simulink model "bike_model_pidTuning"  (R2018b)
settings: Solver=FixedStepAuto  StartTime=0.0  StopTime=sim_time  FixedStep=Ts_IMU  MaxStep=Ts  RelTol=1e-3
values from neighbouring files (symbols this model uses):
  a_compFilter = b_compFilter - 0.77    (= 0.325)    [configuration.m]
  b_compFilter = 1.095    [configuration.m]
  b_real = 1.095    [configuration.m]
  direct_control = 1    [configuration.m]
  IMU_height_real = 0.45    [configuration.m]
  initial_states = [deg2rad(-2) deg2rad(0) deg2rad(0)]    [configuration.m]
  input_velocity = 3    [configuration.m]
  lambda_compFilter = deg2rad(70)    [configuration.m]
  lambda_real = deg2rad(70)    [configuration.m]
  look_ahead = 0    [configuration.m]
  parameters_compFilter = [g h_compFilter b_compFilter a_compFilter lambda_compFilter c_compFilter]    [configuration.m]
  parameters_f_b_real = [m_frame_real m_box_real h_frame_real h_box_real a_frame_real a_box_real c_frame_real c_box_real b_frame_real b_box_real l_frame_real l_box_real]    [configuration.m]
  parameters_real = [g h_real b_real a_real lambda_real c_real]    [configuration.m]
  plant_model = 1    [configuration.m]
  Ts = 0.04    [configuration.m]
  Ts_IMU = 0.04    [configuration.m]
undefined symbols (not defined in the file or in its folder): cumulative_dist_along_path, curvature, DiscIntNeverNeededParam, initial_x, initial_y, lqr_gains, path_x, path_y, sys_con, sys_dis, velocity_lqr
libraries: simulink x20, dspsigops x2
(part 1 of 2)
settings Model: Creator=Boaz Ash  LastModifiedBy=maximef
settings DebuggingCC: UnconnectedInputMsg=none  UnconnectedOutputMsg=none  UnconnectedLineMsg=none  LibraryContextMissingDiagnostic=none
settings SFSimCC: SimUseLocalCustomCode=off
settings RTWCC: RTWUseLocalCustomCode=off

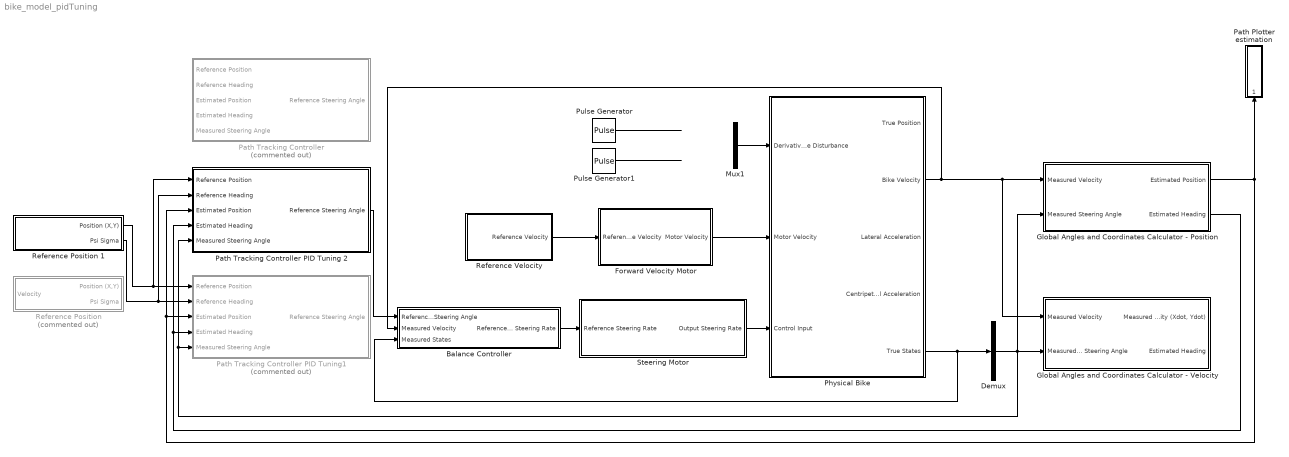
== system bike_model_pidTuning ==
  Balance Controller : Subsystem  TreatAsAtomicUnit=on  SystemSampleTime=Ts
  Demux : Demux  Outputs=3
  Forward Velocity Motor : Subsystem
  Global Angles and Coordinates Calculator - Position : Subsystem  SystemSampleTime=Ts
  Global Angles and Coordinates Calculator - Velocity : Subsystem  SystemSampleTime=Ts
  Mux1 : Mux  Inputs=3
  Path Plotter estimation : Subsystem  SystemSampleTime=Ts
  Path Tracking Controller : Subsystem  Commented=on
  Path Tracking Controller PID Tuning 2 : Subsystem
  Path Tracking Controller PID Tuning1 : Subsystem  Commented=on
  Physical Bike : Subsystem
  Pulse Generator : DiscretePulseGenerator  PulseType=Time based  Amplitude=pi/36  Period=100  PhaseDelay=1
  Pulse Generator1 : DiscretePulseGenerator  PulseType=Time based  Amplitude=-deg2rad(30)  Period=10  PulseWidth=10  PhaseDelay=1
  "Reference Position " : Subsystem  Commented=on
  Reference Position 1 : Subsystem
  "Reference Velocity " : Subsystem
  Steering Motor : Subsystem
  wires:
  Pulse Generator/1 -> ?
  Pulse Generator1/1 -> ?
  Physical Bike/2(Bike Velocity) -> Balance Controller/2(Measured Velocity), Global Angles and Coordinates Calculator - Velocity/1(Measured Velocity), Global Angles and Coordinates Calculator - Position/1(Measured Velocity)
  Reference Position 1/1(Position (X,Y)) -> Path Tracking Controller PID Tuning 2/1(Reference Position), Path Tracking Controller PID Tuning1/1(Reference Position)
  Path Tracking Controller PID Tuning 2/1(Reference Steering Angle) -> Balance Controller/1(Reference Steering Angle)
  Forward Velocity Motor/1(Motor Velocity) -> Physical Bike/2(Motor Velocity)
  Reference Position 1/2(Psi Sigma) -> Path Tracking Controller PID Tuning 2/2(Reference Heading), Path Tracking Controller PID Tuning1/2(Reference Heading)
  "Reference Velocity "/1(Reference Velocity) -> Forward Velocity Motor/1(Reference Velocity)
  Steering Motor/1(Output Steering Rate) -> Physical Bike/3(Control Input)
  Balance Controller/1(Reference Steering Rate) -> Steering Motor/1(Reference Steering Rate)
  Physical Bike/5(True States) -> Balance Controller/3(Measured States), Demux/1
  Global Angles and Coordinates Calculator - Position/2(Estimated Heading) -> Path Tracking Controller PID Tuning 2/4(Estimated Heading), Path Tracking Controller PID Tuning1/4(Estimated Heading)
  Demux/2 -> Global Angles and Coordinates Calculator - Velocity/2("Measured Steering Angle "), Global Angles and Coordinates Calculator - Position/2(Measured Steering Angle), Path Tracking Controller PID Tuning 2/5(Measured Steering Angle), Path Tracking Controller PID Tuning1/5(Measured Steering Angle)
  Mux1/1 -> Physical Bike/1(Derivative Disturbance)
  Global Angles and Coordinates Calculator - Position/1(Estimated Position) -> Path Plotter estimation/1(Position), Path Tracking Controller PID Tuning 2/3(Estimated Position), Path Tracking Controller PID Tuning1/3(Estimated Position)

== system bike_model_pidTuning/Balance Controller ==
  Reference Steering Angle : Inport
  Measured Velocity : Inport  Port=2
  Measured States : Inport  Port=3
  LQR Controller : Subsystem  TreatAsAtomicUnit=on  SystemSampleTime=Ts
  Reference States : Subsystem  SystemSampleTime=Ts
  Sum : Sum  Inputs=|+-
  To Workspace : ToWorkspace  VariableName=states_measured  SaveFormat=Timeseries  SampleTime=-1
  Reference Steering Rate : Outport
  wires:
  Reference States/1(Reference States) -> Sum/1
  Sum/1 -> LQR Controller/2(State Error)
  LQR Controller/1(Calculated Input) -> Reference Steering Rate/1
  Reference Steering Angle/1 -> Reference States/2(Delta Ref)
  Measured Velocity/1 -> Reference States/1(Velocity), LQR Controller/1(Velocity)
  Measured States/1 -> To Workspace/1, Sum/2

== system bike_model_pidTuning/Forward Velocity Motor ==
  note: Add limit for acceleration/deceleration
      | Add min speed of 1.69 m/s (3600 rpm motor speed) limitation
      | Add min speed of 8.20 m/s (18000 rpm motor speed) limitation
      | Add deadband and delay
  Reference Velocity : Inport
  Motor Velocity : Outport
  wires:
  Reference Velocity/1 -> Motor Velocity/1

== system bike_model_pidTuning/Global Angles and Coordinates Calculator - Position ==
  note: True Steering
      | Angle
  Measured Velocity : Inport
  Measured Steering Angle : Inport  Port=2
  Gain1 : Gain  Gain=sin(lambda_compFilter)
  Measured Bike Angles to Global Angles : Subsystem
  Measured Global Angles to Global Coordinates : Subsystem
  Sum : Sum  Inputs=++|
  Estimated Position : Outport
  Estimated Heading : Outport  Port=2
  wires:
  Measured Bike Angles to Global Angles/1(Psi) -> Sum/2, Measured Global Angles to Global Coordinates/2(Psi)
  Gain1/1 -> Measured Bike Angles to Global Angles/2(Measured Steering Angle)
  Sum/1 -> Estimated Heading/1
  Measured Bike Angles to Global Angles/2(Beta) -> Sum/1, Measured Global Angles to Global Coordinates/3(Beta)
  Measured Global Angles to Global Coordinates/1("Position (X, Y)") -> Estimated Position/1
  Measured Velocity/1 -> Measured Global Angles to Global Coordinates/1(Velocity), Measured Bike Angles to Global Angles/1(Velocity)
  Measured Steering Angle/1 -> Gain1/1

== system bike_model_pidTuning/Global Angles and Coordinates Calculator - Velocity ==
  Measured Velocity : Inport
  "Measured Steering Angle " : Inport  Port=2
  Discrete-Time Integrator : DiscreteIntegrator  SampleTime=-1  ICPrevOutput=DiscIntNeverNeededParam  ICPrevScaledInput=DiscIntNeverNeededParam
  Gain1 : Gain  Gain=sin(lambda_compFilter)
  Measured Bike Angles to Global Angles : Subsystem
  Measured Global Angles to Global Coordinates : Subsystem
  Sum : Sum  Inputs=++|
  To Workspace1 : ToWorkspace  VariableName=pos_vel_int  SaveFormat=Timeseries  SampleTime=-1
  "Measured Velocity (Xdot, Ydot)" : Outport
  Estimated Heading : Outport  Port=2
  wires:
  "Measured Steering Angle "/1 -> Gain1/1
  Measured Bike Angles to Global Angles/1(Psi) -> Sum/2, Measured Global Angles to Global Coordinates/2(Psi)
  Gain1/1 -> Measured Bike Angles to Global Angles/2(Measured Steering Angle)
  Sum/1 -> Estimated Heading/1
  Measured Bike Angles to Global Angles/2(Beta) -> Measured Global Angles to Global Coordinates/3(Beta), Sum/1
  Measured Velocity/1 -> Measured Bike Angles to Global Angles/1(Velocity), Measured Global Angles to Global Coordinates/1(Velocity)
  Measured Global Angles to Global Coordinates/1("Velocity (Xdot, Ydot)") -> "Measured Velocity (Xdot, Ydot)"/1, Discrete-Time Integrator/1
  Discrete-Time Integrator/1 -> To Workspace1/1

== system bike_model_pidTuning/Path Plotter estimation ==
  Position : Inport
  Demux : Demux  Outputs=2
  To Workspace : ToWorkspace  VariableName=X_BIKE_estim  SaveFormat=Timeseries  SampleTime=Ts
  To Workspace1 : ToWorkspace  VariableName=Y_BIKE_estim  SaveFormat=Timeseries  SampleTime=Ts
  XY Graph : simulink/Sinks/XY Graph  Commented=on  xmin=min(path_x)-5  xmax=max(path_x)+5  ymin=min(path_y)-5  ymax=max(path_y)+5  st=-1
  wires:
  Demux/1 -> XY Graph/1, To Workspace/1  "X"
  Demux/2 -> XY Graph/2, To Workspace1/1  "Y"
  Position/1 -> Demux/1

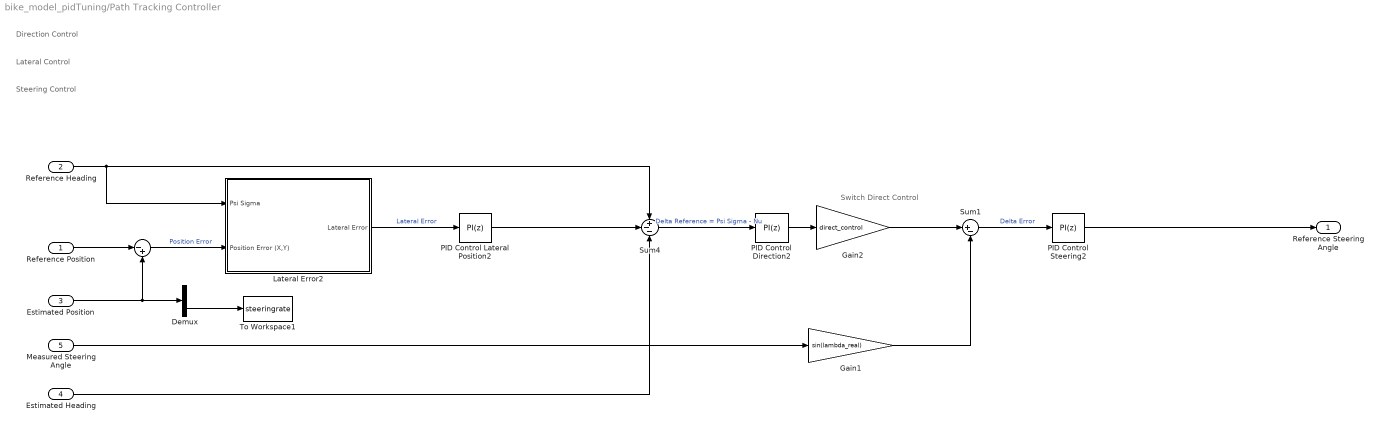
== system bike_model_pidTuning/Path Tracking Controller ==
  note: Direction Control
  note: Lateral Control
  note: Steering Control
  note: Switch Direct Control
  Reference Position : Inport
  Reference Heading : Inport  Port=2
  Estimated Position : Inport  Port=3
  Estimated Heading : Inport  Port=4
  Measured Steering Angle : Inport  Port=5
  " " : Sum  Inputs=|-+
  Demux : Demux  Outputs=2
  Gain1 : Gain  Gain=sin(lambda_real)
  Gain2 : Gain  Gain=direct_control
  Lateral Error2 : Subsystem  SystemSampleTime=Ts
  PID Control Lateral Position2 : simulink/Continuous/PID Controller  Controller=PI  Form=Parallel  TimeDomain=Discrete-time  SampleTime=Ts  IntegratorMethod=Forward Euler  FilterMethod=Forward Euler  ControllerParametersSource=internal  P=0.0465435246389258  I=0.000115580509653549  D=0  UseFilter=on  N=100  TunerSelectOption=Transfer Function Based (PID Tuner App)  InitialConditionSource=internal  InitialConditionForIntegrator=0  InitialConditionForFilter=0  DifferentiatorICPrevScaledInput=0  ExternalReset=none  TrackingMode=off  Kt=1  LimitOutput=off  UpperSaturationLimit=inf  LowerSaturationLimit=-inf  LinearizeAsGain=on  AntiWindupMode=none  Kb=1  POutMin=[]  POutMax=[]  IOutMin=[]  IOutMax=[]  DOutMin=[]  DOutMax=[]  NOutMin=[]  NOutMax=[]  SumOutMin=[]  SumOutMax=[]  SaturationOutMin=[]  SaturationOutMax=[]  PParamMin=[]  PParamMax=[]  IParamMin=[]  IParamMax=[]  DParamMin=[]  DParamMax=[]  NParamMin=[]  NParamMax=[]  KbParamMin=[]  KbParamMax=[]  KtParamMin=[]  KtParamMax=[]  KbOutMin=[]  KbOutMax=[]  KtOutMin=[]  KtOutMax=[]  IntegratorOutMin=[]  IntegratorOutMax=[]  FilterOutMin=[]  FilterOutMax=[]  SumI1OutMin=[]  SumI1OutMax=[]  SumI2OutMin=[]  SumI2OutMax=[]  SumI3OutMin=[]  SumI3OutMax=[]  SumI4OutMin=[]  SumI4OutMax=[]  SumDOutMin=[]  SumDOutMax=[]  DifferentiatorOutMin=[]  DifferentiatorOutMax=[]  FilterDiffOutCoefMin=[]  FilterDiffOutCoefMax=[]  ReciprocalOutMin=[]  ReciprocalOutMax=[]  SumDenOutMin=[]  SumDenOutMax=[]  SumNumOutMin=[]  SumNumOutMax=[]  DivideOutMin=[]  DivideOutMax=[]  IntegratorContinuousStateAttributes=''  IntegratorStateMustResolveToSignalObject=off  IntegratorRTWStateStorageClass=Auto  FilterContinuousStateAttributes=''  FilterStateMustResolveToSignalObject=off  FilterRTWStateStorageClass=Auto  ParallelPVariant=InternalParameters  IdealPVariant=Disabled  IVariant=InternalParameters  DVariant=Disabled  IntegratorVariant=Discrete  SatVariant=Disabled  AWVariant=Passthrough  PCopyVariant=Disabled  TRVariant=Disabled  FdbkBlocksVariant=Forward  IdealPFdbkVariant=Disabled  SatFdbkVariant=Disabled  DerivativeFilterVariant=Disabled  NVariant=Disabled  NCopyVariant=Disabled_SignalSpec  FilterICVariant=Disabled  IntegratorICVariant=InternalICs  ExternalResetVariant=Disabled  TRSumVariant=Passthrough  SumFdbkVariant=Disabled  SumVariant=Sum_PI
  PID Control Direction2 : simulink/Continuous/PID Controller  Controller=PI  Form=Parallel  TimeDomain=Discrete-time  SampleTime=Ts  IntegratorMethod=Forward Euler  FilterMethod=Forward Euler  ControllerParametersSource=internal  P=0.126067479140802  I=0.000739995118675849  D=0  UseFilter=on  N=100  TunerSelectOption=Transfer Function Based (PID Tuner App)  InitialConditionSource=internal  InitialConditionForIntegrator=0  InitialConditionForFilter=0  DifferentiatorICPrevScaledInput=0  ExternalReset=none  TrackingMode=off  Kt=1  LimitOutput=off  UpperSaturationLimit=inf  LowerSaturationLimit=-inf  LinearizeAsGain=on  AntiWindupMode=none  Kb=1  POutMin=[]  POutMax=[]  IOutMin=[]  IOutMax=[]  DOutMin=[]  DOutMax=[]  NOutMin=[]  NOutMax=[]  SumOutMin=[]  SumOutMax=[]  SaturationOutMin=[]  SaturationOutMax=[]  PParamMin=[]  PParamMax=[]  IParamMin=[]  IParamMax=[]  DParamMin=[]  DParamMax=[]  NParamMin=[]  NParamMax=[]  KbParamMin=[]  KbParamMax=[]  KtParamMin=[]  KtParamMax=[]  KbOutMin=[]  KbOutMax=[]  KtOutMin=[]  KtOutMax=[]  IntegratorOutMin=[]  IntegratorOutMax=[]  FilterOutMin=[]  FilterOutMax=[]  SumI1OutMin=[]  SumI1OutMax=[]  SumI2OutMin=[]  SumI2OutMax=[]  SumI3OutMin=[]  SumI3OutMax=[]  SumI4OutMin=[]  SumI4OutMax=[]  SumDOutMin=[]  SumDOutMax=[]  DifferentiatorOutMin=[]  DifferentiatorOutMax=[]  FilterDiffOutCoefMin=[]  FilterDiffOutCoefMax=[]  ReciprocalOutMin=[]  ReciprocalOutMax=[]  SumDenOutMin=[]  SumDenOutMax=[]  SumNumOutMin=[]  SumNumOutMax=[]  DivideOutMin=[]  DivideOutMax=[]  IntegratorContinuousStateAttributes=''  IntegratorStateMustResolveToSignalObject=off  IntegratorRTWStateStorageClass=Auto  FilterContinuousStateAttributes=''  FilterStateMustResolveToSignalObject=off  FilterRTWStateStorageClass=Auto  ParallelPVariant=InternalParameters  IdealPVariant=Disabled  IVariant=InternalParameters  DVariant=Disabled  IntegratorVariant=Discrete  SatVariant=Disabled  AWVariant=Passthrough  PCopyVariant=Disabled  TRVariant=Disabled  FdbkBlocksVariant=Forward  IdealPFdbkVariant=Disabled  SatFdbkVariant=Disabled  DerivativeFilterVariant=Disabled  NVariant=Disabled  NCopyVariant=Disabled_SignalSpec  FilterICVariant=Disabled  IntegratorICVariant=InternalICs  ExternalResetVariant=Disabled  TRSumVariant=Passthrough  SumFdbkVariant=Disabled  SumVariant=Sum_PI
  PID Control Steering2 : simulink/Continuous/PID Controller  Controller=PI  Form=Parallel  TimeDomain=Discrete-time  SampleTime=Ts  IntegratorMethod=Forward Euler  FilterMethod=Forward Euler  ControllerParametersSource=internal  P=0.219020351848633  I=0.4510120195392  D=0  UseFilter=on  N=100  TunerSelectOption=Transfer Function Based (PID Tuner App)  InitialConditionSource=internal  InitialConditionForIntegrator=0  InitialConditionForFilter=0  DifferentiatorICPrevScaledInput=0  ExternalReset=none  TrackingMode=off  Kt=1  LimitOutput=off  UpperSaturationLimit=inf  LowerSaturationLimit=-inf  LinearizeAsGain=on  AntiWindupMode=none  Kb=1  POutMin=[]  POutMax=[]  IOutMin=[]  IOutMax=[]  DOutMin=[]  DOutMax=[]  NOutMin=[]  NOutMax=[]  SumOutMin=[]  SumOutMax=[]  SaturationOutMin=[]  SaturationOutMax=[]  PParamMin=[]  PParamMax=[]  IParamMin=[]  IParamMax=[]  DParamMin=[]  DParamMax=[]  NParamMin=[]  NParamMax=[]  KbParamMin=[]  KbParamMax=[]  KtParamMin=[]  KtParamMax=[]  KbOutMin=[]  KbOutMax=[]  KtOutMin=[]  KtOutMax=[]  IntegratorOutMin=[]  IntegratorOutMax=[]  FilterOutMin=[]  FilterOutMax=[]  SumI1OutMin=[]  SumI1OutMax=[]  SumI2OutMin=[]  SumI2OutMax=[]  SumI3OutMin=[]  SumI3OutMax=[]  SumI4OutMin=[]  SumI4OutMax=[]  SumDOutMin=[]  SumDOutMax=[]  DifferentiatorOutMin=[]  DifferentiatorOutMax=[]  FilterDiffOutCoefMin=[]  FilterDiffOutCoefMax=[]  ReciprocalOutMin=[]  ReciprocalOutMax=[]  SumDenOutMin=[]  SumDenOutMax=[]  SumNumOutMin=[]  SumNumOutMax=[]  DivideOutMin=[]  DivideOutMax=[]  IntegratorContinuousStateAttributes=''  IntegratorStateMustResolveToSignalObject=off  IntegratorRTWStateStorageClass=Auto  FilterContinuousStateAttributes=''  FilterStateMustResolveToSignalObject=off  FilterRTWStateStorageClass=Auto  ParallelPVariant=InternalParameters  IdealPVariant=Disabled  IVariant=InternalParameters  DVariant=Disabled  IntegratorVariant=Discrete  SatVariant=Disabled  AWVariant=Passthrough  PCopyVariant=Disabled  TRVariant=Disabled  FdbkBlocksVariant=Forward  IdealPFdbkVariant=Disabled  SatFdbkVariant=Disabled  DerivativeFilterVariant=Disabled  NVariant=Disabled  NCopyVariant=Disabled_SignalSpec  FilterICVariant=Disabled  IntegratorICVariant=InternalICs  ExternalResetVariant=Disabled  TRSumVariant=Passthrough  SumFdbkVariant=Disabled  SumVariant=Sum_PI
  Sum1 : Sum  Inputs=|+-
  Sum4 : Sum  Inputs=+--
  To Workspace1 : ToWorkspace  VariableName=steeringrate  SaveFormat=Timeseries  SampleTime=Ts
  Reference Steering Angle : Outport
  wires:
  PID Control Steering2/1 -> Reference Steering Angle/1
  Measured Steering Angle/1 -> Gain1/1
  Sum1/1 -> PID Control Steering2/1  "Delta Error"
  Gain1/1 -> Sum1/2
  Sum4/1 -> PID Control Direction2/1  "Delta Reference = Psi Sigma - Nu"
  Estimated Heading/1 -> Sum4/3
  PID Control Direction2/1 -> Gain2/1
  Gain2/1 -> Sum1/1
  Reference Heading/1 -> Sum4/1, Lateral Error2/1(Psi Sigma)
  Reference Position/1 -> " "/1
  Estimated Position/1 -> " "/2, Demux/1
  Lateral Error2/1(Lateral Error) -> PID Control Lateral Position2/1  "Lateral Error"
  " "/1 -> Lateral Error2/2(Position Error (X,Y))  "Position Error"
  PID Control Lateral Position2/1 -> Sum4/2
  Demux/2 -> To Workspace1/1

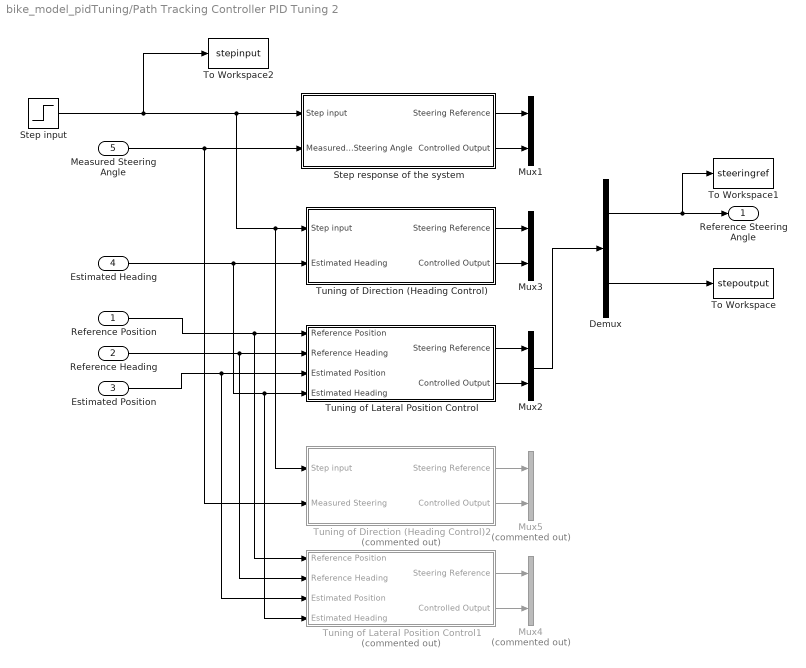
== system bike_model_pidTuning/Path Tracking Controller PID Tuning 2 ==
  Reference Position : Inport
  Reference Heading : Inport  Port=2
  Estimated Position : Inport  Port=3
  Estimated Heading : Inport  Port=4
  Measured Steering Angle : Inport  Port=5
  Demux : Demux  Outputs=2
  Mux1 : Mux  Inputs=2
  Mux2 : Mux  Inputs=2
  Mux3 : Mux  Inputs=2
  Mux4 : Mux  Commented=on  Inputs=2
  Mux5 : Mux  Commented=on  Inputs=2
  Step input : Step  Time=30  After=deg2rad(2)  SampleTime=0
  Step response of the system : Subsystem
  To Workspace : ToWorkspace  VariableName=stepoutput  SaveFormat=Timeseries  SampleTime=-1
  To Workspace1 : ToWorkspace  VariableName=steeringref  SaveFormat=Timeseries  SampleTime=-1
  To Workspace2 : ToWorkspace  VariableName=stepinput  SaveFormat=Timeseries  SampleTime=-1
  Tuning of Direction (Heading Control) : Subsystem
  Tuning of Direction (Heading Control)2 : Subsystem  Commented=on
  Tuning of Lateral Position Control : Subsystem
  Tuning of Lateral Position Control1 : Subsystem  Commented=on
  Reference Steering Angle : Outport
  wires:
  Measured Steering Angle/1 -> Tuning of Direction (Heading Control)2/2(Measured Steering), Step response of the system/2(Measured Steering Angle)
  Estimated Heading/1 -> Tuning of Lateral Position Control1/4(Estimated Heading), Tuning of Lateral Position Control/4(Estimated Heading), Tuning of Direction (Heading Control)/2(Estimated Heading)
  Demux/2 -> To Workspace/1
  Demux/1 -> To Workspace1/1, Reference Steering Angle/1
  Step response of the system/1(Steering Reference) -> Mux1/1
  Step response of the system/2(Controlled Output) -> Mux1/2
  Tuning of Lateral Position Control/1(Steering Reference) -> Mux2/1
  Tuning of Direction (Heading Control)/2(Controlled Output) -> Mux3/2
  Tuning of Direction (Heading Control)/1(Steering Reference) -> Mux3/1
  Tuning of Lateral Position Control/2(Controlled Output) -> Mux2/2
  Mux2/1 -> Demux/1
  Reference Heading/1 -> Tuning of Lateral Position Control1/2(Reference Heading), Tuning of Lateral Position Control/2(Reference Heading)
  Estimated Position/1 -> Tuning of Lateral Position Control1/3(Estimated Position), Tuning of Lateral Position Control/3(Estimated Position)
  Reference Position/1 -> Tuning of Lateral Position Control1/1(Reference Position), Tuning of Lateral Position Control/1(Reference Position)
  Step input/1 -> Tuning of Direction (Heading Control)2/1(Step input), Tuning of Direction (Heading Control)/1(Step input), Step response of the system/1(Step input), To Workspace2/1
  Tuning of Direction (Heading Control)2/2(Controlled Output) -> Mux5/2
  Tuning of Direction (Heading Control)2/1(Steering Reference) -> Mux5/1
  Tuning of Lateral Position Control1/2(Controlled Output) -> Mux4/2
  Tuning of Lateral Position Control1/1(Steering Reference) -> Mux4/1

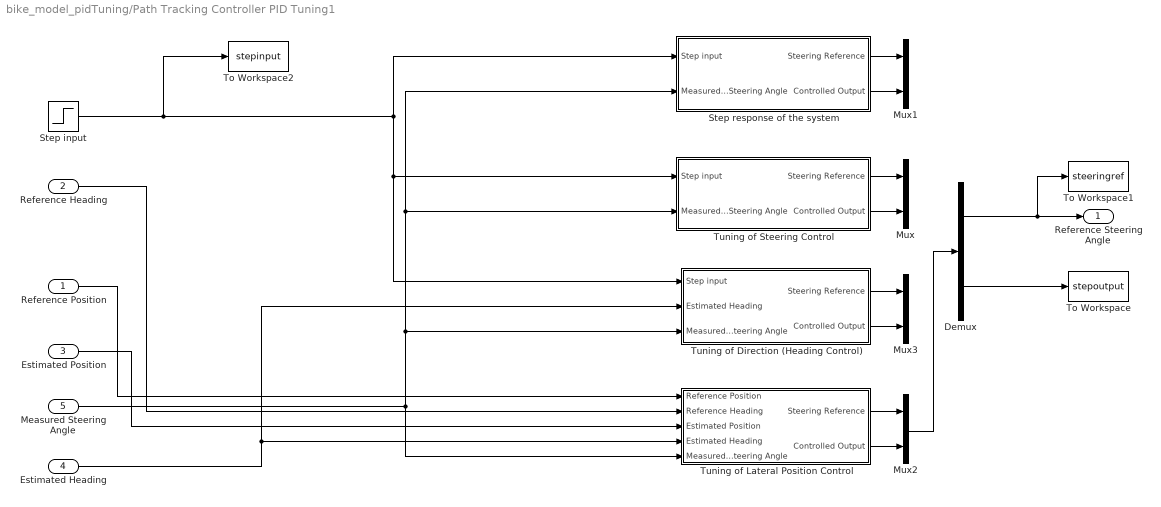
== system bike_model_pidTuning/Path Tracking Controller PID Tuning1 ==
  Reference Position : Inport
  Reference Heading : Inport  Port=2
  Estimated Position : Inport  Port=3
  Estimated Heading : Inport  Port=4
  Measured Steering Angle : Inport  Port=5
  Demux : Demux  Outputs=2
  Mux{,1..3} (4 alike) : Mux  Inputs=2
  Step input : Step  Time=15  After=deg2rad(2)  SampleTime=0
  Step response of the system : Subsystem
  To Workspace : ToWorkspace  VariableName=stepoutput  SaveFormat=Timeseries  SampleTime=-1
  To Workspace1 : ToWorkspace  VariableName=steeringref  SaveFormat=Timeseries  SampleTime=-1
  To Workspace2 : ToWorkspace  VariableName=stepinput  SaveFormat=Timeseries  SampleTime=-1
  Tuning of Direction (Heading Control) : Subsystem
  Tuning of Lateral Position Control : Subsystem
  Tuning of Steering Control : Subsystem
  Reference Steering Angle : Outport
  wires:
  Measured Steering Angle/1 -> Step response of the system/2(Measured Steering Angle), Tuning of Steering Control/2(Measured Steering Angle), Tuning of Direction (Heading Control)/3(Measured Steering Angle), Tuning of Lateral Position Control/5(Measured Steering Angle)
  Estimated Heading/1 -> Tuning of Direction (Heading Control)/2(Estimated Heading), Tuning of Lateral Position Control/4(Estimated Heading)
  Demux/2 -> To Workspace/1
  Demux/1 -> To Workspace1/1, Reference Steering Angle/1
  Tuning of Steering Control/1(Steering Reference) -> Mux/1
  Tuning of Steering Control/2(Controlled Output) -> Mux/2
  Step response of the system/1(Steering Reference) -> Mux1/1
  Step response of the system/2(Controlled Output) -> Mux1/2
  Tuning of Lateral Position Control/1(Steering Reference) -> Mux2/1
  Tuning of Direction (Heading Control)/2(Controlled Output) -> Mux3/2
  Tuning of Direction (Heading Control)/1(Steering Reference) -> Mux3/1
  Tuning of Lateral Position Control/2(Controlled Output) -> Mux2/2
  Mux2/1 -> Demux/1
  Reference Heading/1 -> Tuning of Lateral Position Control/2(Reference Heading)
  Estimated Position/1 -> Tuning of Lateral Position Control/3(Estimated Position)
  Reference Position/1 -> Tuning of Lateral Position Control/1(Reference Position)
  Step input/1 -> To Workspace2/1, Step response of the system/1(Step input), Tuning of Direction (Heading Control)/1(Step input), Tuning of Steering Control/1(Step input)

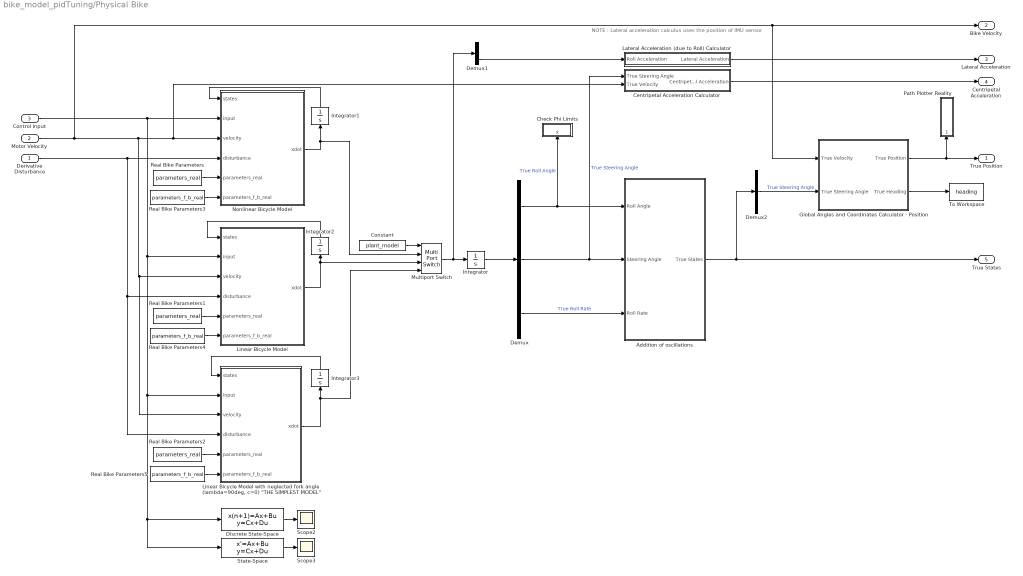
== system bike_model_pidTuning/Physical Bike ==
  note: NOTE : Lateral acceleration calculus uses the position of IMU sensor
  Derivative Disturbance : Inport
  Motor Velocity : Inport  Port=2
  Control Input : Inport  Port=3
  " Addition of oscillations" : Subsystem  SystemSampleTime=Ts
  Centripetal Acceleration Calculator : Subsystem
  Check Phi Limits : Subsystem  TreatAsAtomicUnit=on  SystemSampleTime=Ts
  Constant : Constant  Value=plant_model
  Demux : Demux  Outputs=3
  Demux1 : Demux  Outputs=3
  Demux2 : Demux  Outputs=3
  Discrete State-Space : DiscreteStateSpace  A=sys_dis.A  B=sys_dis.B  C=eye(3,3)  D=zeros(3,1)  SampleTime=Ts_IMU
  Global Angles and Coordinates Calculator - Position : Subsystem  SystemSampleTime=Ts
  Integrator{,1..3} (4 alike) : Integrator  InitialCondition=initial_states
  Lateral Acceleration (due to Roll) Calculator : Subsystem
  Linear Bicycle Model : MATLAB Function  TreatAsAtomicUnit=on
  "Linear Bicycle Model with neglected fork angle (lambda=90deg, c=0) \"THE SIMPLEST MODEL\"" : MATLAB Function  TreatAsAtomicUnit=on
  Multiport Switch : MultiPortSwitch
  Nonlinear Bicycle Model : MATLAB Function  TreatAsAtomicUnit=on
  Path Plotter Reality : Subsystem  SystemSampleTime=Ts
  Real Bike Parameters : Constant  Value=parameters_real
  Real Bike Parameters1 : Constant  Value=parameters_real
  Real Bike Parameters2 : Constant  Value=parameters_real
  Real Bike Parameters3 : Constant  Value=parameters_f_b_real
  Real Bike Parameters4 : Constant  Value=parameters_f_b_real
  Real Bike Parameters5 : Constant  Value=parameters_f_b_real
  Scope2 : Scope
  Scope3 : Scope
  State-Space : StateSpace  A=sys_con.A  B=sys_con.B  C=eye(3,3)  D=zeros(3,1)  InitialCondition=0
  To Workspace : ToWorkspace  VariableName=heading  SaveFormat=Timeseries  SampleTime=Ts
  True Position : Outport
  Bike Velocity : Outport  Port=2
  Lateral Acceleration : Outport  Port=3
  Centripetal Acceleration : Outport  Port=4
  True States : Outport  Port=5
  wires:
  Real Bike Parameters5/1 -> "Linear Bicycle Model with neglected fork angle (lambda=90deg, c=0) \"THE SIMPLEST MODEL\""/6(parameters_f_b_real)
  Demux/2 -> Centripetal Acceleration Calculator/1(True Steering Angle), " Addition of oscillations"/2(Steering Angle)  "True Steering Angle"
  Control Input/1 -> Nonlinear Bicycle Model/2(input), State-Space/1, Discrete State-Space/1, "Linear Bicycle Model with neglected fork angle (lambda=90deg, c=0) \"THE SIMPLEST MODEL\""/2(input), Linear Bicycle Model/2(input)
  Integrator1/1 -> Nonlinear Bicycle Model/1(states)
  Real Bike Parameters3/1 -> Nonlinear Bicycle Model/6(parameters_f_b_real)
  Constant/1 -> Multiport Switch/1
  Real Bike Parameters2/1 -> "Linear Bicycle Model with neglected fork angle (lambda=90deg, c=0) \"THE SIMPLEST MODEL\""/5(parameters_real)
  State-Space/1 -> Scope3/1
  Discrete State-Space/1 -> Scope2/1
  Integrator/1 -> Demux/1
  Demux/1 -> Check Phi Limits/1(x), " Addition of oscillations"/1(Roll Angle)  "True Roll Angle"
  Real Bike Parameters1/1 -> Linear Bicycle Model/5(parameters_real)
  Centripetal Acceleration Calculator/1(Centripetal Acceleration) -> Centripetal Acceleration/1
  Nonlinear Bicycle Model/1(xdot) -> Integrator1/1, Multiport Switch/2
  Demux1/3 -> Lateral Acceleration (due to Roll) Calculator/1(Roll Acceleration)
  Linear Bicycle Model/1(xdot) -> Integrator2/1, Multiport Switch/3
  Derivative Disturbance/1 -> "Linear Bicycle Model with neglected fork angle (lambda=90deg, c=0) \"THE SIMPLEST MODEL\""/4(disturbance), Linear Bicycle Model/4(disturbance), Nonlinear Bicycle Model/4(disturbance)
  Real Bike Parameters/1 -> Nonlinear Bicycle Model/5(parameters_real)
  "Linear Bicycle Model with neglected fork angle (lambda=90deg, c=0) \"THE SIMPLEST MODEL\""/1(xdot) -> Integrator3/1, Multiport Switch/4
  Multiport Switch/1 -> Demux1/1, Integrator/1
  Lateral Acceleration (due to Roll) Calculator/1(Lateral Acceleration) -> Lateral Acceleration/1
  Integrator3/1 -> "Linear Bicycle Model with neglected fork angle (lambda=90deg, c=0) \"THE SIMPLEST MODEL\""/1(states)
  Integrator2/1 -> Linear Bicycle Model/1(states)
  Motor Velocity/1 -> Global Angles and Coordinates Calculator - Position/1(True Velocity), Bike Velocity/1, Centripetal Acceleration Calculator/2(True Velocity), Nonlinear Bicycle Model/3(velocity), "Linear Bicycle Model with neglected fork angle (lambda=90deg, c=0) \"THE SIMPLEST MODEL\""/3(velocity), Linear Bicycle Model/3(velocity)
  Real Bike Parameters4/1 -> Linear Bicycle Model/6(parameters_f_b_real)
  Demux/3 -> " Addition of oscillations"/3(Roll Rate)  "True Roll Rate"
  " Addition of oscillations"/1(True States) -> Demux2/1, True States/1
  Demux2/2 -> Global Angles and Coordinates Calculator - Position/2(True Steering Angle)  "True Steering Angle"
  Global Angles and Coordinates Calculator - Position/1(True Position) -> True Position/1, Path Plotter Reality/1(Position)
  Global Angles and Coordinates Calculator - Position/2(True Heading) -> To Workspace/1

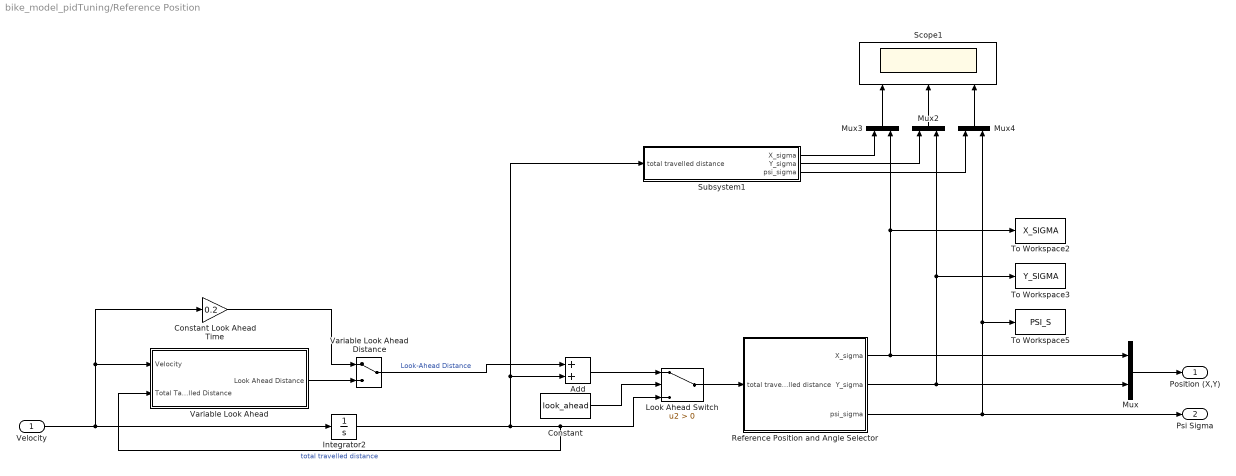
== system bike_model_pidTuning/Reference Position  ==
  Velocity : Inport
  Add : Sum
  Constant : Constant  Value=look_ahead
  Constant Look Ahead Time : Gain  Gain=0.2
  Integrator2 : Integrator
  Look Ahead Switch : Switch  Criteria=u2 > Threshold
  Mux{,2..4} (4 alike) : Mux  Inputs=2
  Reference Position and Angle Selector : Subsystem
  Scope1 : Scope  NumInputPorts=3
  Subsystem1 : Subsystem
  To Workspace2 : ToWorkspace  VariableName=X_SIGMA  SaveFormat=Timeseries  SampleTime=Ts
  To Workspace3 : ToWorkspace  VariableName=Y_SIGMA  SaveFormat=Timeseries  SampleTime=Ts
  To Workspace5 : ToWorkspace  VariableName=PSI_S  SaveFormat=Timeseries  SampleTime=Ts
  Variable Look Ahead Distance : ManualSwitch
  Variable Look Ahead : Subsystem
  Position (X,Y) : Outport
  Psi Sigma : Outport  Port=2
  wires:
  Constant Look Ahead Time/1 -> Variable Look Ahead Distance/1
  Reference Position and Angle Selector/3(psi_sigma) -> To Workspace5/1, Mux4/2, Psi Sigma/1
  Mux3/1 -> Scope1/1
  Subsystem1/3(psi_sigma) -> Mux4/1
  Mux2/1 -> Scope1/2
  Mux4/1 -> Scope1/3
  Velocity/1 -> Integrator2/1, Constant Look Ahead Time/1, Variable Look Ahead/1(Velocity)
  Add/1 -> Look Ahead Switch/1
  Reference Position and Angle Selector/2(Y_sigma) -> To Workspace3/1, Mux2/2, Mux/2
  Look Ahead Switch/1 -> Reference Position and Angle Selector/1(total travelled distance)
  Subsystem1/2(Y_sigma) -> Mux2/1
  Integrator2/1 -> Variable Look Ahead/2(Total Tavelled Distance), Look Ahead Switch/3, Subsystem1/1(total travelled distance), Add/2  "total travelled distance"
  Subsystem1/1(X_sigma) -> Mux3/1
  Reference Position and Angle Selector/1(X_sigma) -> Mux3/2, To Workspace2/1, Mux/1
  Variable Look Ahead Distance/1 -> Add/1  "Look-Ahead Distance"
  Constant/1 -> Look Ahead Switch/2
  Mux/1 -> Position (X,Y)/1
  Variable Look Ahead/1(Look Ahead Distance) -> Variable Look Ahead Distance/2

== system bike_model_pidTuning/Reference Position 1 ==
  Constant : Constant  Value=0
  Mux : Mux  Inputs=2
  Ramp : simulink/Sources/Ramp  slope=3  start=0  InitialOutput=0
  Step2 : Step  Time=15  After=0.1  SampleTime=0
  To Workspace2 : ToWorkspace  VariableName=X_SIGMA  SaveFormat=Timeseries  SampleTime=Ts
  To Workspace3 : ToWorkspace  VariableName=Y_SIGMA  SaveFormat=Timeseries  SampleTime=Ts
  Position (X,Y) : Outport
  Psi Sigma : Outport  Port=2
  wires:
  Mux/1 -> Position (X,Y)/1
  Ramp/1 -> To Workspace2/1, Mux/1
  Step2/1 -> Mux/2, To Workspace3/1

== system bike_model_pidTuning/Reference Velocity  ==
  Constant Velocity : Constant  Value=input_velocity
  Reference Velocity : Outport
  wires:
  Constant Velocity/1 -> Reference Velocity/1

== system bike_model_pidTuning/Steering Motor ==
  Reference Steering Rate : Inport
  To Workspace : ToWorkspace  VariableName=calculated_input  SaveFormat=Timeseries  SampleTime=Ts
  To Workspace1 : ToWorkspace  VariableName=realised_input  SaveFormat=Timeseries  SampleTime=Ts
  Output Steering Rate : Outport
  wires:
  Reference Steering Rate/1 -> Output Steering Rate/1, To Workspace1/1, To Workspace/1

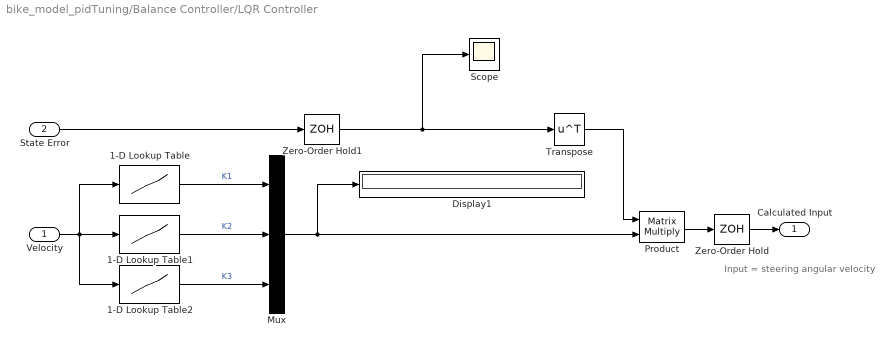
== system bike_model_pidTuning/Balance Controller/LQR Controller ==
  note: Input = steering angular velocity
  Velocity : Inport
  State Error : Inport  Port=2
  1-D Lookup Table : Lookup_n-D  NumberOfTableDimensions=1  BreakpointsForDimension1=velocity_lqr  BreakpointsForDimension2=velocity_lqr  BreakpointsForDimension3=velocity_lqr  BreakpointsForDimension4=velocity_lqr  Table=lqr_gains(:,1)  InternalRulePriority=Speed  RndMeth=Simplest  InputSameDT=on
  1-D Lookup Table1 : Lookup_n-D  NumberOfTableDimensions=1  BreakpointsForDimension1=velocity_lqr  BreakpointsForDimension2=velocity_lqr  BreakpointsForDimension3=velocity_lqr  BreakpointsForDimension4=velocity_lqr  Table=lqr_gains(:,2)  InternalRulePriority=Speed  RndMeth=Simplest  InputSameDT=on
  1-D Lookup Table2 : Lookup_n-D  NumberOfTableDimensions=1  BreakpointsForDimension1=velocity_lqr  BreakpointsForDimension2=velocity_lqr  BreakpointsForDimension3=velocity_lqr  BreakpointsForDimension4=velocity_lqr  Table=lqr_gains(:,3)  InternalRulePriority=Speed  RndMeth=Simplest  InputSameDT=on
  Display1 : Display
  Mux : Mux  Inputs=3
  Product : Product  Multiplication=Matrix(*)
  Scope : Scope
  Transpose : Math  Operator=transpose  SaturateOnIntegerOverflow=on
  Zero-Order Hold : ZeroOrderHold  SampleTime=Ts
  Zero-Order Hold1 : ZeroOrderHold  SampleTime=Ts
  Calculated Input : Outport
  wires:
  1-D Lookup Table/1 -> Mux/1  "K1"
  1-D Lookup Table1/1 -> Mux/2  "K2"
  State Error/1 -> Zero-Order Hold1/1
  Product/1 -> Zero-Order Hold/1
  1-D Lookup Table2/1 -> Mux/3  "K3"
  Velocity/1 -> 1-D Lookup Table2/1, 1-D Lookup Table1/1, 1-D Lookup Table/1
  Mux/1 -> Product/2, Display1/1
  Transpose/1 -> Product/1
  Zero-Order Hold/1 -> Calculated Input/1
  Zero-Order Hold1/1 -> Scope/1, Transpose/1

== system bike_model_pidTuning/Balance Controller/Reference States ==
  Velocity : Inport
  Delta Ref : Inport  Port=2
  Bike Parameters : Constant  Value=parameters_real
  Mux5 : Mux  Inputs=3
  Reference Roll Angle Calculator : MATLAB Function  TreatAsAtomicUnit=on
  Reference States : Outport
  wires:
  Bike Parameters/1 -> Reference Roll Angle Calculator/1(parameters_real)
  Delta Ref/1 -> Mux5/2, Reference Roll Angle Calculator/3(delta_ref)
  Reference Roll Angle Calculator/1(phi_ref) -> Mux5/1
  Velocity/1 -> Reference Roll Angle Calculator/2(velocity)
  Mux5/1 -> Reference States/1

== system bike_model_pidTuning/Global Angles and Coordinates Calculator - Position/Measured Bike Angles to Global Angles ==
  Velocity : Inport
  Measured Steering Angle : Inport  Port=2
  " Bike Parameters Model " : Constant  Value=parameters_compFilter
  Integrator : Integrator
  MATLAB Function : MATLAB Function  TreatAsAtomicUnit=on
  Psi : Outport
  Beta : Outport  Port=2
  wires:
  MATLAB Function/2(beta) -> Beta/1
  MATLAB Function/1(psi_d) -> Integrator/1
  Integrator/1 -> Psi/1
  " Bike Parameters Model "/1 -> MATLAB Function/2(parameters_model)
  Measured Steering Angle/1 -> MATLAB Function/3(delta)
  Velocity/1 -> MATLAB Function/1(v)

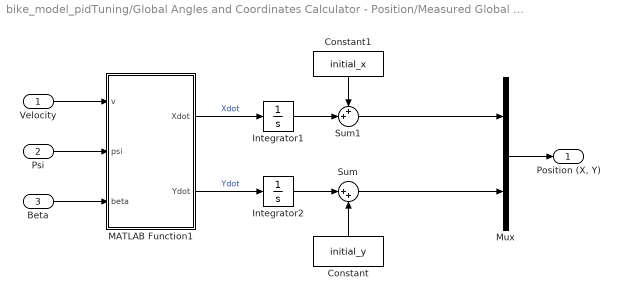
== system bike_model_pidTuning/Global Angles and Coordinates Calculator - Position/Measured Global Angles to Global Coordinates ==
  Velocity : Inport
  Psi : Inport  Port=2
  Beta : Inport  Port=3
  Constant : Constant  Value=initial_y
  Constant1 : Constant  Value=initial_x
  Integrator1 : Integrator
  Integrator2 : Integrator
  MATLAB Function1 : MATLAB Function  TreatAsAtomicUnit=on
  Mux : Mux  Inputs=2
  Sum : Sum  Inputs=|++
  Sum1 : Sum  Inputs=++|
  "Position (X, Y)" : Outport
  wires:
  MATLAB Function1/2(Ydot) -> Integrator2/1  "Ydot"
  MATLAB Function1/1(Xdot) -> Integrator1/1  "Xdot"
  Psi/1 -> MATLAB Function1/2(psi)
  Beta/1 -> MATLAB Function1/3(beta)
  Velocity/1 -> MATLAB Function1/1(v)
  Integrator2/1 -> Sum/1
  Constant/1 -> Sum/2
  Sum/1 -> Mux/2
  Integrator1/1 -> Sum1/2
  Sum1/1 -> Mux/1
  Constant1/1 -> Sum1/1
  Mux/1 -> "Position (X, Y)"/1

== system bike_model_pidTuning/Global Angles and Coordinates Calculator - Velocity/Measured Bike Angles to Global Angles ==
  note: Verification of the equivalence of the calculus for Beta estimation
  Velocity : Inport
  Measured Steering Angle : Inport  Port=2
  Gain : Gain  Gain=1/b_compFilter
  Integrator : Integrator
  MATLAB Function : MATLAB Function  TreatAsAtomicUnit=on
  Multiply : Product
  Parameters : Constant  Value=parameters_compFilter
  Scope : Scope  NumInputPorts=2
  Tan : Trigonometry  Operator=tan
  Psi : Outport
  Beta : Outport  Port=2
  wires:
  Integrator/1 -> Psi/1
  MATLAB Function/1(psi_d) -> Scope/1, Integrator/1
  Measured Steering Angle/1 -> Tan/1, MATLAB Function/3(delta)
  Parameters/1 -> MATLAB Function/2(parameters_model)
  Velocity/1 -> Multiply/1, MATLAB Function/1(v)
  MATLAB Function/2(beta) -> Beta/1
  Tan/1 -> Multiply/2
  Multiply/1 -> Gain/1
  Gain/1 -> Scope/2

== system bike_model_pidTuning/Global Angles and Coordinates Calculator - Velocity/Measured Global Angles to Global Coordinates ==
  Velocity : Inport
  Psi : Inport  Port=2
  Beta : Inport  Port=3
  MATLAB Function1 : MATLAB Function  TreatAsAtomicUnit=on
  Mux1 : Mux  Inputs=2
  "Velocity (Xdot, Ydot)" : Outport
  wires:
  MATLAB Function1/2(Ydot) -> Mux1/2  "Ydot"
  MATLAB Function1/1(Xdot) -> Mux1/1  "Xdot"
  Psi/1 -> MATLAB Function1/2(psi)
  Beta/1 -> MATLAB Function1/3(beta)
  Velocity/1 -> MATLAB Function1/1(v)
  Mux1/1 -> "Velocity (Xdot, Ydot)"/1

== system bike_model_pidTuning/Path Tracking Controller/Lateral Error2 ==
  Psi Sigma : Inport
  Position Error (X,Y) : Inport  Port=2
  Cos : Trigonometry  Operator=cos
  Demux : Demux  Outputs=2
  Product : Product
  Product1 : Product
  Sin : Trigonometry
  Sum : Sum  Inputs=+-|
  To Workspace4 : ToWorkspace  VariableName=LAT_ERR  SaveFormat=Timeseries  SampleTime=Ts
  Lateral Error : Outport
  wires:
  Cos/1 -> Product/2
  Sin/1 -> Product1/1
  Psi Sigma/1 -> Cos/1, Sin/1
  Product1/1 -> Sum/2
  Product/1 -> Sum/1
  Sum/1 -> To Workspace4/1, Lateral Error/1  "Lateral Error"
  Demux/1 -> Product1/2  "X Position Error"
  Demux/2 -> Product/1  "Y Position Error"
  Position Error (X,Y)/1 -> Demux/1

== system bike_model_pidTuning/Path Tracking Controller PID Tuning 2/Step response of the system ==
  Step input : Inport
  Measured Steering Angle : Inport  Port=2
  Gain : Gain  Gain=2/3
  Steering Reference : Outport
  Controlled Output : Outport  Port=2
  wires:
  Step input/1 -> Gain/1
  Measured Steering Angle/1 -> Controlled Output/1
  Gain/1 -> Steering Reference/1

== system bike_model_pidTuning/Path Tracking Controller PID Tuning 2/Tuning of Direction (Heading Control) ==
  Step input : Inport
  Estimated Heading : Inport  Port=2
  PID Control Direction2 : simulink/Continuous/PID Controller  Controller=PID  Form=Parallel  TimeDomain=Discrete-time  SampleTime=Ts  IntegratorMethod=Forward Euler  FilterMethod=Forward Euler  ControllerParametersSource=internal  P=0.5  I=0.5  D=0.1  UseFilter=off  N=100  TunerSelectOption=Transfer Function Based (PID Tuner App)  InitialConditionSource=internal  InitialConditionForIntegrator=0  InitialConditionForFilter=0  DifferentiatorICPrevScaledInput=0  ExternalReset=none  TrackingMode=off  Kt=1  LimitOutput=off  UpperSaturationLimit=inf  LowerSaturationLimit=-inf  LinearizeAsGain=on  AntiWindupMode=none  Kb=1  POutMin=[]  POutMax=[]  IOutMin=[]  IOutMax=[]  DOutMin=[]  DOutMax=[]  NOutMin=[]  NOutMax=[]  SumOutMin=[]  SumOutMax=[]  SaturationOutMin=[]  SaturationOutMax=[]  PParamMin=[]  PParamMax=[]  IParamMin=[]  IParamMax=[]  DParamMin=[]  DParamMax=[]  NParamMin=[]  NParamMax=[]  KbParamMin=[]  KbParamMax=[]  KtParamMin=[]  KtParamMax=[]  KbOutMin=[]  KbOutMax=[]  KtOutMin=[]  KtOutMax=[]  IntegratorOutMin=[]  IntegratorOutMax=[]  FilterOutMin=[]  FilterOutMax=[]  SumI1OutMin=[]  SumI1OutMax=[]  SumI2OutMin=[]  SumI2OutMax=[]  SumI3OutMin=[]  SumI3OutMax=[]  SumI4OutMin=[]  SumI4OutMax=[]  SumDOutMin=[]  SumDOutMax=[]  DifferentiatorOutMin=[]  DifferentiatorOutMax=[]  FilterDiffOutCoefMin=[]  FilterDiffOutCoefMax=[]  ReciprocalOutMin=[]  ReciprocalOutMax=[]  SumDenOutMin=[]  SumDenOutMax=[]  SumNumOutMin=[]  SumNumOutMax=[]  DivideOutMin=[]  DivideOutMax=[]  IntegratorContinuousStateAttributes=''  IntegratorStateMustResolveToSignalObject=off  IntegratorRTWStateStorageClass=Auto  FilterContinuousStateAttributes=''  FilterStateMustResolveToSignalObject=off  FilterRTWStateStorageClass=Auto  ParallelPVariant=InternalParameters  IdealPVariant=Disabled  IVariant=InternalParameters  DVariant=InternalParameters  IntegratorVariant=Discrete  SatVariant=Disabled  AWVariant=Passthrough  PCopyVariant=Disabled  TRVariant=Disabled  FdbkBlocksVariant=Forward  IdealPFdbkVariant=Disabled  SatFdbkVariant=Disabled  DerivativeFilterVariant=Differentiator  NVariant=Passthrough  NCopyVariant=Disabled_SignalSpec  FilterICVariant=InternalICsDifferentiator  IntegratorICVariant=InternalICs  ExternalResetVariant=Disabled  TRSumVariant=Passthrough  SumFdbkVariant=Disabled  SumVariant=Sum_PID
  Sum4 : Sum  Inputs=+--
  Steering Reference : Outport
  Controlled Output : Outport  Port=2
  wires:
  Estimated Heading/1 -> Controlled Output/1, Sum4/3
  Sum4/1 -> PID Control Direction2/1  "Delta Reference = Psi Sigma - Nu"
  Step input/1 -> Sum4/1
  PID Control Direction2/1 -> Steering Reference/1

== system bike_model_pidTuning/Path Tracking Controller PID Tuning 2/Tuning of Direction (Heading Control)2 ==
  Step input : Inport
  Measured Steering : Inport  Port=2
  PID Control Direction2 : simulink/Continuous/PID Controller  Controller=PI  Form=Parallel  TimeDomain=Discrete-time  SampleTime=Ts  IntegratorMethod=Forward Euler  FilterMethod=Forward Euler  ControllerParametersSource=internal  P=0.578359413467721  I=0.617399561418389  D=0  UseFilter=on  N=100  TunerSelectOption=Transfer Function Based (PID Tuner App)  InitialConditionSource=internal  InitialConditionForIntegrator=0  InitialConditionForFilter=0  DifferentiatorICPrevScaledInput=0  ExternalReset=none  TrackingMode=off  Kt=1  LimitOutput=off  UpperSaturationLimit=inf  LowerSaturationLimit=-inf  LinearizeAsGain=on  AntiWindupMode=none  Kb=1  POutMin=[]  POutMax=[]  IOutMin=[]  IOutMax=[]  DOutMin=[]  DOutMax=[]  NOutMin=[]  NOutMax=[]  SumOutMin=[]  SumOutMax=[]  SaturationOutMin=[]  SaturationOutMax=[]  PParamMin=[]  PParamMax=[]  IParamMin=[]  IParamMax=[]  DParamMin=[]  DParamMax=[]  NParamMin=[]  NParamMax=[]  KbParamMin=[]  KbParamMax=[]  KtParamMin=[]  KtParamMax=[]  KbOutMin=[]  KbOutMax=[]  KtOutMin=[]  KtOutMax=[]  IntegratorOutMin=[]  IntegratorOutMax=[]  FilterOutMin=[]  FilterOutMax=[]  SumI1OutMin=[]  SumI1OutMax=[]  SumI2OutMin=[]  SumI2OutMax=[]  SumI3OutMin=[]  SumI3OutMax=[]  SumI4OutMin=[]  SumI4OutMax=[]  SumDOutMin=[]  SumDOutMax=[]  DifferentiatorOutMin=[]  DifferentiatorOutMax=[]  FilterDiffOutCoefMin=[]  FilterDiffOutCoefMax=[]  ReciprocalOutMin=[]  ReciprocalOutMax=[]  SumDenOutMin=[]  SumDenOutMax=[]  SumNumOutMin=[]  SumNumOutMax=[]  DivideOutMin=[]  DivideOutMax=[]  IntegratorContinuousStateAttributes=''  IntegratorStateMustResolveToSignalObject=off  IntegratorRTWStateStorageClass=Auto  FilterContinuousStateAttributes=''  FilterStateMustResolveToSignalObject=off  FilterRTWStateStorageClass=Auto  ParallelPVariant=InternalParameters  IdealPVariant=Disabled  IVariant=InternalParameters  DVariant=Disabled  IntegratorVariant=Discrete  SatVariant=Disabled  AWVariant=Passthrough  PCopyVariant=Disabled  TRVariant=Disabled  FdbkBlocksVariant=Forward  IdealPFdbkVariant=Disabled  SatFdbkVariant=Disabled  DerivativeFilterVariant=Disabled  NVariant=Disabled  NCopyVariant=Disabled_SignalSpec  FilterICVariant=Disabled  IntegratorICVariant=InternalICs  ExternalResetVariant=Disabled  TRSumVariant=Passthrough  SumFdbkVariant=Disabled  SumVariant=Sum_PI
  Sum4 : Sum  Inputs=+--
  Transfer Fcn : TransferFcn  Numerator=[1 0]  Denominator=[a_compFilter/b_compFilter input_velocity/a_compFilter]
  Steering Reference : Outport
  Controlled Output : Outport  Port=2
  wires:
  Step input/1 -> Transfer Fcn/1
  PID Control Direction2/1 -> Steering Reference/1
  Measured Steering/1 -> Controlled Output/1, Sum4/3
  Transfer Fcn/1 -> Sum4/1
  Sum4/1 -> PID Control Direction2/1

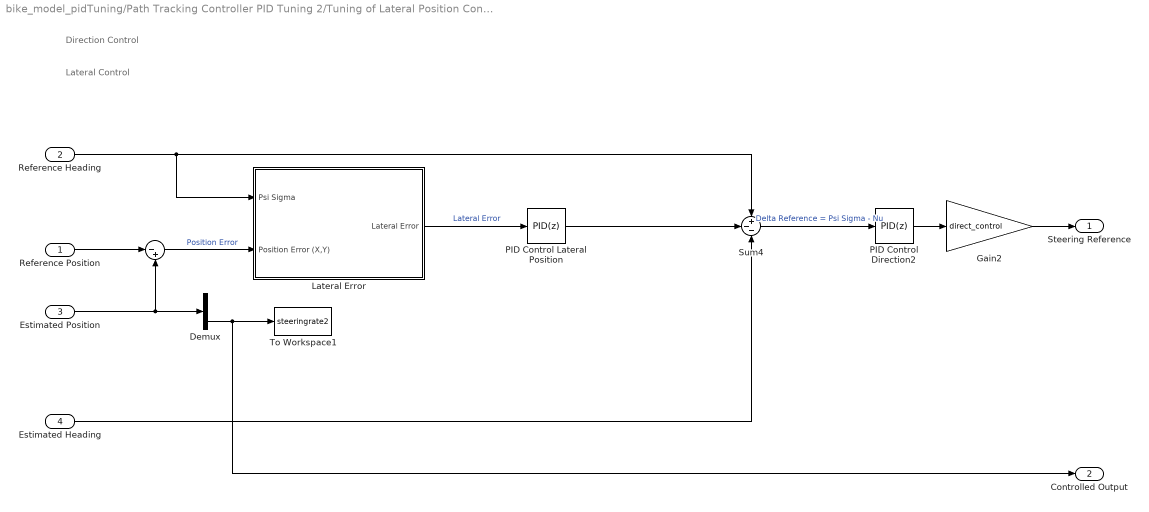
== system bike_model_pidTuning/Path Tracking Controller PID Tuning 2/Tuning of Lateral Position Control ==
  note: Direction Control
  note: Lateral Control
  Reference Position : Inport
  Reference Heading : Inport  Port=2
  Estimated Position : Inport  Port=3
  Estimated Heading : Inport  Port=4
  " " : Sum  Inputs=|-+
  Demux : Demux  Outputs=2
  Gain2 : Gain  Gain=direct_control
  Lateral Error : Subsystem  SystemSampleTime=Ts
  PID Control Lateral Position : simulink/Continuous/PID Controller  Controller=PID  Form=Parallel  TimeDomain=Discrete-time  SampleTime=Ts  IntegratorMethod=Forward Euler  FilterMethod=Forward Euler  ControllerParametersSource=internal  P=0.15  I=0  D=0  UseFilter=on  N=38.085941813801  TunerSelectOption=Transfer Function Based (PID Tuner App)  InitialConditionSource=internal  InitialConditionForIntegrator=0  InitialConditionForFilter=0  DifferentiatorICPrevScaledInput=0  ExternalReset=none  TrackingMode=off  Kt=1  LimitOutput=off  UpperSaturationLimit=inf  LowerSaturationLimit=-inf  LinearizeAsGain=on  AntiWindupMode=none  Kb=1  POutMin=[]  POutMax=[]  IOutMin=[]  IOutMax=[]  DOutMin=[]  DOutMax=[]  NOutMin=[]  NOutMax=[]  SumOutMin=[]  SumOutMax=[]  SaturationOutMin=[]  SaturationOutMax=[]  PParamMin=[]  PParamMax=[]  IParamMin=[]  IParamMax=[]  DParamMin=[]  DParamMax=[]  NParamMin=[]  NParamMax=[]  KbParamMin=[]  KbParamMax=[]  KtParamMin=[]  KtParamMax=[]  KbOutMin=[]  KbOutMax=[]  KtOutMin=[]  KtOutMax=[]  IntegratorOutMin=[]  IntegratorOutMax=[]  FilterOutMin=[]  FilterOutMax=[]  SumI1OutMin=[]  SumI1OutMax=[]  SumI2OutMin=[]  SumI2OutMax=[]  SumI3OutMin=[]  SumI3OutMax=[]  SumI4OutMin=[]  SumI4OutMax=[]  SumDOutMin=[]  SumDOutMax=[]  DifferentiatorOutMin=[]  DifferentiatorOutMax=[]  FilterDiffOutCoefMin=[]  FilterDiffOutCoefMax=[]  ReciprocalOutMin=[]  ReciprocalOutMax=[]  SumDenOutMin=[]  SumDenOutMax=[]  SumNumOutMin=[]  SumNumOutMax=[]  DivideOutMin=[]  DivideOutMax=[]  IntegratorContinuousStateAttributes=''  IntegratorStateMustResolveToSignalObject=off  IntegratorRTWStateStorageClass=Auto  FilterContinuousStateAttributes=''  FilterStateMustResolveToSignalObject=off  FilterRTWStateStorageClass=Auto  ParallelPVariant=InternalParameters  IdealPVariant=Disabled  IVariant=InternalParameters  DVariant=InternalParameters  IntegratorVariant=Discrete  SatVariant=Disabled  AWVariant=Passthrough  PCopyVariant=Disabled  TRVariant=Disabled  FdbkBlocksVariant=Forward  IdealPFdbkVariant=Disabled  SatFdbkVariant=Disabled  DerivativeFilterVariant=ForwardEulerFilter  NVariant=InternalParameters  NCopyVariant=Disabled  FilterICVariant=InternalICsFilter  IntegratorICVariant=InternalICs  ExternalResetVariant=Disabled  TRSumVariant=Passthrough  SumFdbkVariant=Disabled  SumVariant=Sum_PID
  PID Control Direction2 : simulink/Continuous/PID Controller  Controller=PID  Form=Parallel  TimeDomain=Discrete-time  SampleTime=Ts  IntegratorMethod=Forward Euler  FilterMethod=Forward Euler  ControllerParametersSource=internal  P=0.6  I=0  D=0  UseFilter=on  N=2.10117245247272  TunerSelectOption=Transfer Function Based (PID Tuner App)  InitialConditionSource=internal  InitialConditionForIntegrator=0  InitialConditionForFilter=0  DifferentiatorICPrevScaledInput=0  ExternalReset=none  TrackingMode=off  Kt=1  LimitOutput=off  UpperSaturationLimit=inf  LowerSaturationLimit=-inf  LinearizeAsGain=on  AntiWindupMode=none  Kb=1  POutMin=[]  POutMax=[]  IOutMin=[]  IOutMax=[]  DOutMin=[]  DOutMax=[]  NOutMin=[]  NOutMax=[]  SumOutMin=[]  SumOutMax=[]  SaturationOutMin=[]  SaturationOutMax=[]  PParamMin=[]  PParamMax=[]  IParamMin=[]  IParamMax=[]  DParamMin=[]  DParamMax=[]  NParamMin=[]  NParamMax=[]  KbParamMin=[]  KbParamMax=[]  KtParamMin=[]  KtParamMax=[]  KbOutMin=[]  KbOutMax=[]  KtOutMin=[]  KtOutMax=[]  IntegratorOutMin=[]  IntegratorOutMax=[]  FilterOutMin=[]  FilterOutMax=[]  SumI1OutMin=[]  SumI1OutMax=[]  SumI2OutMin=[]  SumI2OutMax=[]  SumI3OutMin=[]  SumI3OutMax=[]  SumI4OutMin=[]  SumI4OutMax=[]  SumDOutMin=[]  SumDOutMax=[]  DifferentiatorOutMin=[]  DifferentiatorOutMax=[]  FilterDiffOutCoefMin=[]  FilterDiffOutCoefMax=[]  ReciprocalOutMin=[]  ReciprocalOutMax=[]  SumDenOutMin=[]  SumDenOutMax=[]  SumNumOutMin=[]  SumNumOutMax=[]  DivideOutMin=[]  DivideOutMax=[]  IntegratorContinuousStateAttributes=''  IntegratorStateMustResolveToSignalObject=off  IntegratorRTWStateStorageClass=Auto  FilterContinuousStateAttributes=''  FilterStateMustResolveToSignalObject=off  FilterRTWStateStorageClass=Auto  ParallelPVariant=InternalParameters  IdealPVariant=Disabled  IVariant=InternalParameters  DVariant=InternalParameters  IntegratorVariant=Discrete  SatVariant=Disabled  AWVariant=Passthrough  PCopyVariant=Disabled  TRVariant=Disabled  FdbkBlocksVariant=Forward  IdealPFdbkVariant=Disabled  SatFdbkVariant=Disabled  DerivativeFilterVariant=ForwardEulerFilter  NVariant=InternalParameters  NCopyVariant=Disabled  FilterICVariant=InternalICsFilter  IntegratorICVariant=InternalICs  ExternalResetVariant=Disabled  TRSumVariant=Passthrough  SumFdbkVariant=Disabled  SumVariant=Sum_PID
  Sum4 : Sum  Inputs=+--
  To Workspace1 : ToWorkspace  VariableName=steeringrate2  SaveFormat=Timeseries  SampleTime=Ts
  Steering Reference : Outport
  Controlled Output : Outport  Port=2
  wires:
  PID Control Lateral Position/1 -> Sum4/2
  Reference Heading/1 -> Sum4/1, Lateral Error/1(Psi Sigma)
  Lateral Error/1(Lateral Error) -> PID Control Lateral Position/1  "Lateral Error"
  Reference Position/1 -> " "/1
  Estimated Heading/1 -> Sum4/3
  " "/1 -> Lateral Error/2(Position Error (X,Y))  "Position Error"
  Sum4/1 -> PID Control Direction2/1  "Delta Reference = Psi Sigma - Nu"
  Demux/2 -> Controlled Output/1, To Workspace1/1
  PID Control Direction2/1 -> Gain2/1
  Gain2/1 -> Steering Reference/1
  Estimated Position/1 -> " "/2, Demux/1
